simulink subsystem "atmosphere"  (R2020a)
settings: Solver=VariableStepAuto  StartTime=0.0  StopTime=10.0  RelTol=1e-3
values from neighbouring files (symbols this model uses):
  interpAltitude = placeholder_index_asc    [configure_simulation.m]
  latIndex = placeholder_index_asc    [configure_simulation.m]    (also in get_gfs_data.m = indices{1,2})
  lonIndex = placeholder_index_asc    [configure_simulation.m]    (also in get_gfs_data.m = indices{2,2})
  Mair = molar_mass('air')    [configure_simulation.m]
  pressureVsAltitude = placeholder_datacube    [configure_simulation.m]
  temperatureVsPressure = {placeholder_index_desc, placeholder_datacube}    [configure_simulation.m]
  use_std_atmo = false    [configure_simulation.m]
  uWindVsPressure = {placeholder_index_desc, placeholder_datacube}    [configure_simulation.m]
  vWindVsPressure = {placeholder_index_desc, placeholder_datacube}    [configure_simulation.m]
  zWindVsPressure = {placeholder_index_desc, placeholder_datacube}    [configure_simulation.m]
libraries: aerolibatmos2 x1
settings Model: Creator=Philip  LastModifiedBy=Philip

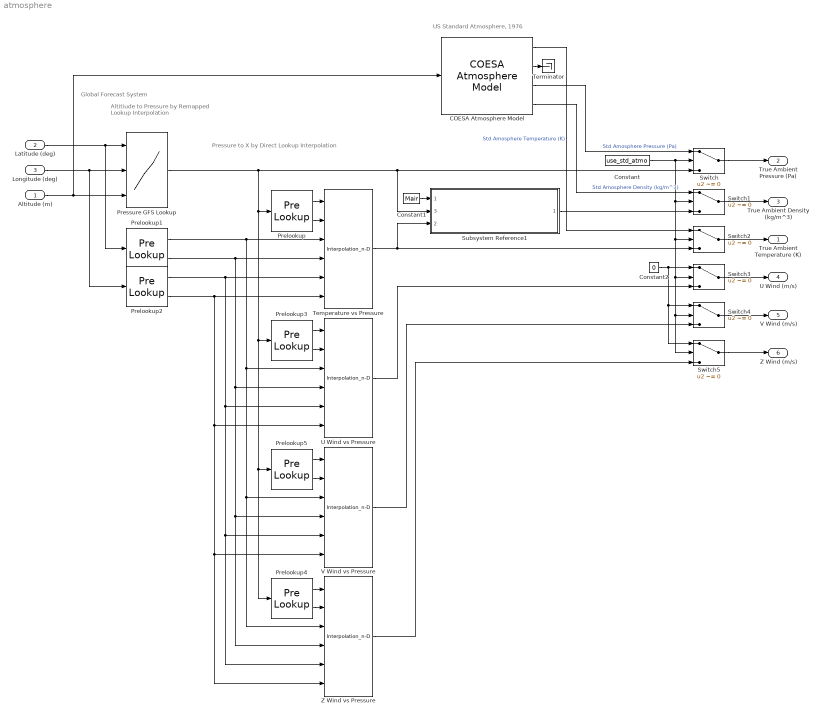
== system atmosphere ==
  note: Global Forecast System
  note: Altitiude to Pressure
      | by Remapped Lookup
      | Interpolation
  note: Pressure to X
      | by Direct Lookup Interpolation
  note: US Standard Atmosphere, 1976
  Altitude (m) : Inport
  Latitude (deg) : Inport  Port=2
  Longitude (deg) : Inport  Port=3
  COESA Atmosphere Model : aerolibatmos2/COESA Atmosphere Model  units=Metric (MKS)  spec=1976 COESA-extended U.S. Standard Atmosphere  model=Profile  profile_var=High temperature  profile_percent=1%  profile_alt=5 km (16404 ft)  envelope_var=High temperature  envelope_percent=1%  action=Warning
  Constant : Constant  Value=use_std_atmo
  Constant1 : Constant  Value=Mair
  Constant2 : Constant  Value=0
  Prelookup : PreLookup  BreakpointsData=flip(temperatureVsPressure{1})
  Prelookup1 : PreLookup  BreakpointsData=latIndex
  Prelookup2 : PreLookup  BreakpointsData=lonIndex
  Prelookup3 : PreLookup  BreakpointsData=flip(uWindVsPressure{1})
  Prelookup4 : PreLookup  BreakpointsData=flip(zWindVsPressure{1})
  Prelookup5 : PreLookup  BreakpointsData=flip(vWindVsPressure{1})
  Pressure GFS Lookup : Lookup_n-D  NumberOfTableDimensions=3  BreakpointsForDimension1=latIndex  BreakpointsForDimension2=lonIndex  BreakpointsForDimension3=interpAltitude  BeginIndexSearchUsingPreviousIndexResult=on  Table=pressureVsAltitude  ExtrapMethod=Clip  UseLastTableValue=on  InternalRulePriority=Speed  OutMin=0  RndMeth=Simplest  InputSameDT=on
  Subsystem Reference1 : Subsystem  ReferencedSubsystem=rho_ideal
      settings: PortSchema="{\"entries\":[{\"content\":{\"sides\":[{\"content\":{\"connectorIds\":[\"In1\",\"In3\",\"In2\"]},\"type\":\"ConnectorPlacement.EquallySpacedRectSide\",\"uuid\":\"735561a8-65a4-40e9-ab18-c9a7e172788e\"},{\"content\":{\"connectorIds\":[\"Out1\"],\"side\":\"RIGHT\"},\"type\":\"ConnectorPlacement.EquallySpacedRectSide\",\"uuid\":\"27a8ea76-56ad-4824-abed-48b3e31af730\"},{\"content\":{\"connectorIds\":[],\"side\":\"TOP\"},\"type\":\"ConnectorPlacement.EquallySpacedRectSide\",\"uuid\":\"f63bc076-3668-4e6d-83e4-3ea5fd7adc29\"}]},\"type\":\"ConnectorPlacement.EquallySpacedConnector\",\"uuid\":\"a3334ca5-08ab-41be-8424-de45103cfacd\"}],\"packageUris\":[\"http://schema.mathworks.com/mf0/Connector/19700101\"],\"version\":\"1.0\"}"
  Switch{,1..5} (6 alike) : Switch  Criteria=u2 ~= 0  Threshold=true
  Temperature vs Pressure : Interpolation_n-D  NumberOfTableDimensions=3  Table=flip(temperatureVsPressure{2},1)  ExtrapMethod=Clip  InternalRulePriority=Speed
      settings: InputPortMap=u0,u1,u2,u3,u4,u5
  Terminator : Terminator
  U Wind vs Pressure : Interpolation_n-D  NumberOfTableDimensions=3  Table=flip(uWindVsPressure{2},1)  ExtrapMethod=Clip  InternalRulePriority=Speed
      settings: InputPortMap=u0,u1,u2,u3,u4,u5
  V Wind vs Pressure : Interpolation_n-D  NumberOfTableDimensions=3  Table=flip(vWindVsPressure{2},1)  ExtrapMethod=Clip  InternalRulePriority=Speed
      settings: InputPortMap=u0,u1,u2,u3,u4,u5
  Z Wind vs Pressure : Interpolation_n-D  NumberOfTableDimensions=3  Table=flip(zWindVsPressure{2},1)  ExtrapMethod=Clip  InternalRulePriority=Speed
      settings: InputPortMap=u0,u1,u2,u3,u4,u5
  True Ambient Temperature (K) : Outport
  True Ambient Pressure (Pa) : Outport  Port=2
  True Ambient Density (kg/m^3) : Outport  Port=3
  U Wind (m/s) : Outport  Port=4
  V Wind (m/s) : Outport  Port=5
  Z Wind (m/s) : Outport  Port=6
  wires:
  Constant2/1 -> Switch5/1, Switch4/1, Switch3/1
  Switch5/1 -> Z Wind (m/s)/1
  Switch4/1 -> V Wind (m/s)/1
  Switch3/1 -> U Wind (m/s)/1
  Switch2/1 -> True Ambient Temperature (K)/1
  Switch1/1 -> True Ambient Density (kg/m^3)/1
  Switch/1 -> True Ambient Pressure (Pa)/1
  Constant/1 -> Switch3/2, Switch5/2, Switch4/2, Switch2/2, Switch1/2, Switch/2
  Longitude (deg)/1 -> Pressure GFS Lookup/2, Prelookup2/1
  Latitude (deg)/1 -> Pressure GFS Lookup/1, Prelookup1/1
  Pressure GFS Lookup/1 -> Switch/3, Subsystem Reference1/3, Prelookup3/1, Prelookup4/1, Prelookup5/1, Prelookup/1
  Constant1/1 -> Subsystem Reference1/1
  Subsystem Reference1/1 -> Switch1/3
  Altitude (m)/1 -> COESA Atmosphere Model/1, Pressure GFS Lookup/3
  COESA Atmosphere Model/2 -> Terminator/1
  COESA Atmosphere Model/3 -> Switch/1  "Std Amosphere Pressure (Pa)"
  COESA Atmosphere Model/4 -> Switch1/1  "Std Amosphere Density (kg/m^3)"
  COESA Atmosphere Model/1 -> Switch2/1  "Std Amosphere Temperature (K)"
  Prelookup/1 -> Temperature vs Pressure/1
  Prelookup/2 -> Temperature vs Pressure/2
  Temperature vs Pressure/1 -> Switch2/3, Subsystem Reference1/2
  Prelookup1/1 -> U Wind vs Pressure/3, V Wind vs Pressure/3, Z Wind vs Pressure/3, Temperature vs Pressure/3
  Prelookup1/2 -> V Wind vs Pressure/4, Z Wind vs Pressure/4, U Wind vs Pressure/4, Temperature vs Pressure/4
  Prelookup2/1 -> U Wind vs Pressure/5, V Wind vs Pressure/5, Z Wind vs Pressure/5, Temperature vs Pressure/5
  Prelookup2/2 -> U Wind vs Pressure/6, V Wind vs Pressure/6, Z Wind vs Pressure/6, Temperature vs Pressure/6
  Prelookup3/1 -> U Wind vs Pressure/1
  Prelookup3/2 -> U Wind vs Pressure/2
  U Wind vs Pressure/1 -> Switch3/3
  V Wind vs Pressure/1 -> Switch4/3
  Prelookup5/1 -> V Wind vs Pressure/1
  Prelookup5/2 -> V Wind vs Pressure/2
  Prelookup4/1 -> Z Wind vs Pressure/1
  Prelookup4/2 -> Z Wind vs Pressure/2
  Z Wind vs Pressure/1 -> Switch5/3
